simulink model "test_pi_gazebo_2023a"  (R2023a)
settings: Solver=FixedStepAuto  StartTime=0.0  StopTime=inf  RelTol=1e-3
undefined symbols (not defined in the file): angular, DiscIntNeverNeededParam, linear
libraries: ros2lib x14, robotcorelib x3, simulink x1
settings Model: Creator=johvany  LastModifiedBy=l15
settings OptimizationCC: EnhancedBackFolding=on  PassReuseOutputArgsThreshold=0  ZeroExternalMemoryAtStartup=off  ZeroInternalMemoryAtStartup=off  MaxStackSize=64  OptimizeBlockOrder=speed  DifferentSizesBufferReuse=on  OptimizationCustomize=off
settings DebuggingCC: ParameterTunabilityLossMsg=error
settings HardwareCC: ProdBitPerLong=64  ProdHWDeviceType=Intel->x86-64 (Linux 64)  UseEmbeddedCoderFeatures=off
settings SFSimCC: MATLABDynamicMemAlloc=off
settings RTWCC: Description=Embedded Coder  SystemTargetFile=ert.tlc  HardwareBoard=Robot Operating System 2 (ROS 2)  TLCOptions="-aInlineSetEventsForThisBaseRateFcn=TLC_FALSE -aSuppressMultiTaskScheduler=TLC_FALSE  -aRateBasedStepFcn=0"  TemplateMakefile=ert_default_tmf  Toolchain=Colcon Tools  TargetLang=C++
settings CodeAppCC: ForceParamTrailComments=on  OperatorAnnotations=on
settings ERTTargetCC: ERTCustomFileBanners=off  CodeInterfacePackaging=C++ class  SupportContinuousTime=on  SupportNonInlinedSFcns=on  RemoveResetFunc=off  ModelStepFunctionPrototypeControlCompliant=off  RootIOFormat=Structure reference

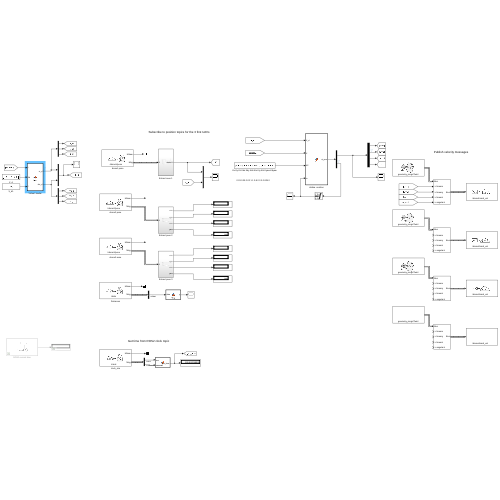
[thumbnail: Simulink's stored preview of the top-level diagram]
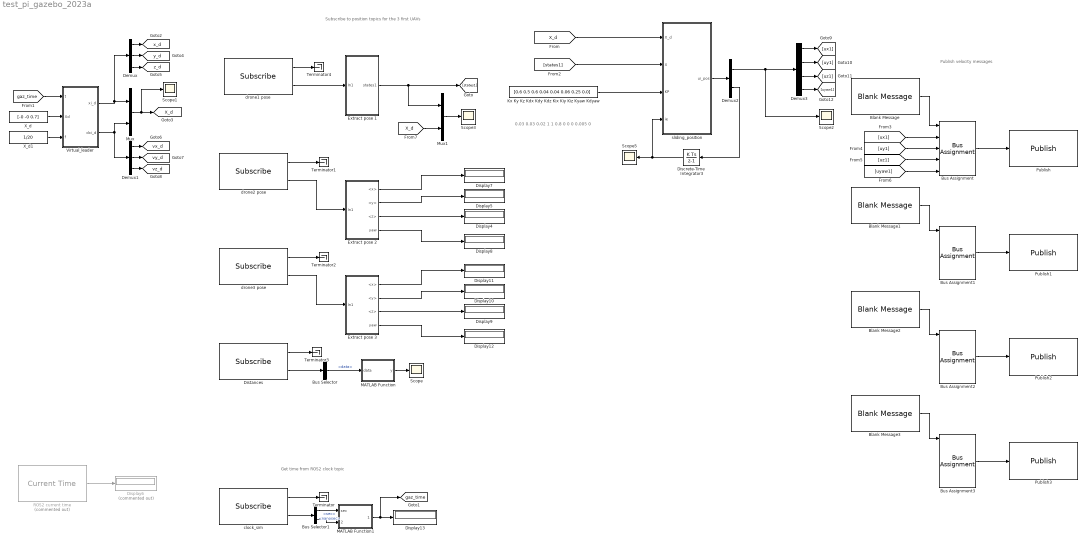
== system test_pi_gazebo_2023a ==
  note: Publish velocity messages
  note: Subscribe to position topics for the 3 first UAVs
  note: Get time from ROS2 clock topic
  note: 0.03 0.03 0.02 1 1 0.8 0 0 0 0.005 0
  Blank Message{,1..3} (4 alike) : ros2lib/Blank Message  messageClass=Message  entityType=geometry_msgs/Twist  messageType=geometry_msgs/Twist  SampleTime=inf
  Bus Assignment{,1..3} (4 alike) : BusAssignment  AssignedSignals=linear.x,linear.y,linear.z,angular.z
  Bus Selector : BusSelector  OutputSignals=data
  Bus Selector1 : BusSelector  OutputSignals=clock.sec,clock.nanosec
  Demux : Demux  Outputs=3
  Demux1 : Demux  Outputs=3
  Demux2 : Demux  Outputs=2
  Demux3 : Demux
  Discrete-Time Integrator3 : DiscreteIntegrator  SampleTime=-1  LimitOutput=on  UpperSaturationLimit=1  LowerSaturationLimit=-1  ICPrevOutput=DiscIntNeverNeededParam  ICPrevScaledInput=DiscIntNeverNeededParam
  Display{4..5,7..13} (9 alike) : Display
      Display13 settings: Decimation=4
  Display6 : Display  Commented=on
  Distances : ros2lib/Subscribe  topicSource=Select from ROS network  topic=/dists  messageType=std_msgs/Float32MultiArray  sampleTime=-1  QOSHistory=Keep last  QOSDepth=1  QOSReliability=Reliable  QOSDurability=Volatile
  Extract pose 1 : Subsystem
  Extract pose 2 : Subsystem
  Extract pose 3 : Subsystem
  Kx Ky Kz Kdx Kdy Kdz Kix Kiy Kiz Kyaw Kdyaw : Constant  Value=[0.6 0.5 0.6 0.04 0.04 0.06 0.25 0.0]
  MATLAB Function : MATLAB Function  TreatAsAtomicUnit=on
  MATLAB Function1 : MATLAB Function  TreatAsAtomicUnit=on
  Mux : Mux  Inputs=2
  Mux1 : Mux  Inputs=2
  Publish : ros2lib/Publish  topicSource=Select from ROS network  topic=/drone1/cmd_vel  messageType=geometry_msgs/Twist  QOSHistory=Keep last  QOSDepth=1  QOSReliability=Reliable  QOSDurability=Volatile
  Publish1 : ros2lib/Publish  topicSource=Select from ROS network  topic=/drone2/cmd_vel  messageType=geometry_msgs/Twist  QOSHistory=Keep last  QOSDepth=1  QOSReliability=Reliable  QOSDurability=Volatile
  Publish2 : ros2lib/Publish  topicSource=Select from ROS network  topic=/drone3/cmd_vel  messageType=geometry_msgs/Twist  QOSHistory=Keep last  QOSDepth=1  QOSReliability=Reliable  QOSDurability=Volatile
  Publish3 : ros2lib/Publish  topicSource=Select from ROS network  topic=/drone4/cmd_vel  messageType=geometry_msgs/Twist  QOSHistory=Keep last  QOSDepth=1  QOSReliability=Reliable  QOSDurability=Volatile
  ROS2 current time : ros2lib/Current Time  Commented=on  OutputFormat=double  SampleTime=-1  ModelName=test_pid_gazebo
  Scope{,1..3,5} (5 alike) : Scope
  Terminator{,1..4} (5 alike) : Terminator
  Virtual_leader : MATLAB Function  TreatAsAtomicUnit=on
  X_d : Constant  Value=[-0 -0 0.7]
  X_d1 : Constant  Value=1/20
  clock_sim : ros2lib/Subscribe  topicSource=Select from ROS network  topic=/clock  messageType=rosgraph_msgs/Clock  sampleTime=-1  QOSHistory=Keep last  QOSDepth=1  QOSReliability=Reliable  QOSDurability=Volatile
  drone1 pose : ros2lib/Subscribe  topicSource=Select from ROS network  topic=/drone1/pose  messageType=geometry_msgs/PoseStamped  sampleTime=-1  QOSHistory=Keep last  QOSDepth=1  QOSReliability=Reliable  QOSDurability=Volatile
  drone2 pose : ros2lib/Subscribe  topicSource=Select from ROS network  topic=/drone2/pose  messageType=geometry_msgs/PoseStamped  sampleTime=-1  QOSHistory=Keep last  QOSDepth=1  QOSReliability=Reliable  QOSDurability=Volatile
  drone3 pose : ros2lib/Subscribe  topicSource=Select from ROS network  topic=/drone3/pose  messageType=geometry_msgs/PoseStamped  sampleTime=-1  QOSHistory=Keep last  QOSDepth=1  QOSReliability=Reliable  QOSDurability=Volatile
  sliding_position : MATLAB Function  TreatAsAtomicUnit=on
  tag scope: X_d=global, gaz_time=global, vx_d=global, vy_d=global, vz_d=global, x_d=global, y_d=global, z_d=global
  wires:
  clock_sim/1 -> Terminator/1
  ROS2 current time/1 -> Display6/1
  Extract pose 2/3(<z>) -> Display4/1
  drone2 pose/2 -> Extract pose 2/1(In1)
  Extract pose 2/1(<x>) -> Display7/1
  Extract pose 2/4(yaw) -> Display8/1
  Extract pose 2/2(<y>) -> Display5/1
  drone2 pose/1 -> Terminator1/1
  Extract pose 3/3(<z>) -> Display9/1
  drone3 pose/2 -> Extract pose 3/1(In1)
  Extract pose 3/1(<x>) -> Display11/1
  Extract pose 3/4(yaw) -> Display12/1
  Extract pose 3/2(<y>) -> Display10/1
  drone3 pose/1 -> Terminator2/1
  Blank Message/1 -> Bus Assignment/1
  Bus Assignment/1 -> Publish/1
  Blank Message1/1 -> Bus Assignment1/1
  Bus Assignment1/1 -> Publish1/1
  Blank Message2/1 -> Bus Assignment2/1
  Bus Assignment2/1 -> Publish2/1
  Blank Message3/1 -> Bus Assignment3/1
  Bus Assignment3/1 -> Publish3/1
  Distances/1 -> Terminator3/1
  Distances/2 -> Bus Selector/1
  Bus Selector/1 -> MATLAB Function/1(data)  "<data>"
  MATLAB Function/1(y) -> Scope/1
  sliding_position/1(ui_pos) -> Demux2/1
  Discrete-Time Integrator3/1 -> Scope5/1, sliding_position/4(ie)
  [states1] -> sliding_position/2(X)
  Demux2/2 -> Discrete-Time Integrator3/1
  [X_d] -> sliding_position/1(X_d)
  clock_sim/2 -> Bus Selector1/1
  Bus Selector1/1 -> MATLAB Function1/1(sec)  "<sec>"
  Bus Selector1/2 -> MATLAB Function1/2(nanosec)  "<nanosec>"
  Demux1/1 -> [vx_d]
  Demux1/3 -> [vz_d]
  Demux/1 -> [x_d]
  Demux/2 -> [y_d]
  Virtual_leader/2(dxi_d) -> Mux/2, Demux1/1
  Mux/1 -> Scope1/1, [X_d]
  Demux1/2 -> [vy_d]
  [gaz_time] -> Virtual_leader/1(t)
  Demux/3 -> [z_d]
  Virtual_leader/1(xi_d) -> Demux/1, Mux/1
  drone1 pose/1 -> Terminator4/1
  drone1 pose/2 -> Extract pose 1/1(In1)
  MATLAB Function1/1(gaz_time) -> [gaz_time], Display13/1
  Extract pose 1/1(states1) -> Mux1/1, [states1]
  Kx Ky Kz Kdx Kdy Kdz Kix Kiy Kiz Kyaw Kdyaw/1 -> sliding_position/3(KP)
  Demux2/1 -> Scope2/1, Demux3/1
  Demux3/1 -> [ux1]
  Demux3/3 -> [uz1]
  Demux3/2 -> [uy1]
  [ux1] -> Bus Assignment/2
  [uy1] -> Bus Assignment/3
  [uz1] -> Bus Assignment/4
  [uyaw1] -> Bus Assignment/5
  X_d/1 -> Virtual_leader/2(Xd)
  Demux3/4 -> [uyaw1]
  [X_d] -> Mux1/2
  Mux1/1 -> Scope3/1
  X_d1/1 -> Virtual_leader/3(f)

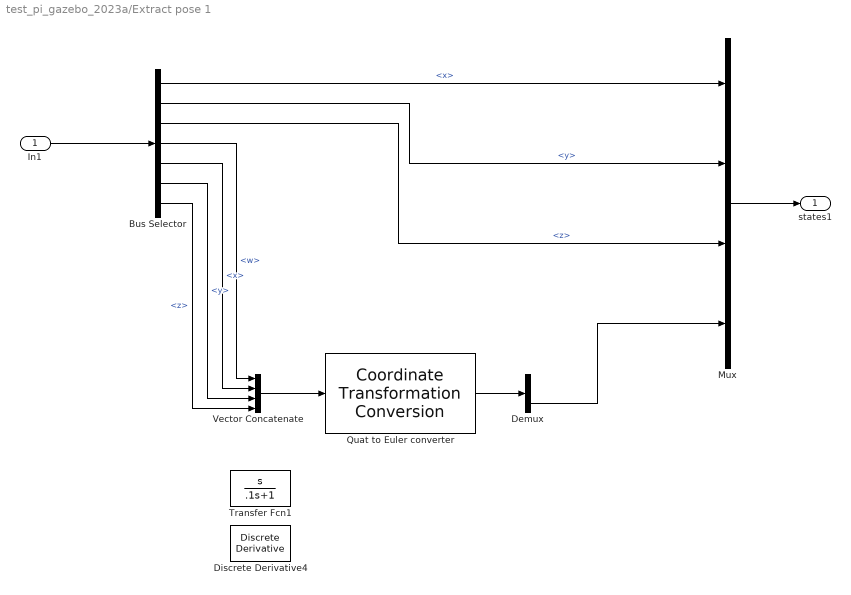
== system test_pi_gazebo_2023a/Extract pose 1 ==
  In1 : Inport
  Bus Selector : BusSelector  OutputSignals=pose.position.x,pose.position.y,pose.position.z,pose.orientation.w,pose.orientation.x,pose.orientation.y,pose.orientation.z
  Demux : Demux  Outputs=3
  Discrete Derivative4 : simulink/Discrete/Discrete Derivative  gainval=1.0  ICPrevScaledInput=0.0  OutMin=[]  OutMax=[]  OutDataType=fixdt(1, 16)  OutScaling=2^-10  DoSatur=off
  Mux : Mux
  Quat to Euler converter : robotcorelib/Coordinate Transformation Conversion  InputRepresentation=Quaternion  InputEulerSequence=ZYX  ShowTrVecInputPort=on  OutputRepresentation=Euler Angles  OutputEulerSequence=XYZ  ShowTrVecOutputPort=on  SimulateUsing=Interpreted execution
      settings: LibrarySourceBlock=roslib/Utilities/Coordinate Transformation Conversion
  Transfer Fcn1 : TransferFcn  Numerator=[1 0]  Denominator=[.1 1]
  Vector Concatenate : Concatenate  NumInputs=4
  states1 : Outport
  wires:
  Bus Selector/5 -> Vector Concatenate/2  "<x>"
  Quat to Euler converter/1 -> Demux/1
  Demux/3 -> Mux/4
  Bus Selector/6 -> Vector Concatenate/3  "<y>"
  Bus Selector/1 -> Mux/1  "<x>"
  Bus Selector/7 -> Vector Concatenate/4  "<z>"
  Vector Concatenate/1 -> Quat to Euler converter/1
  In1/1 -> Bus Selector/1
  Bus Selector/4 -> Vector Concatenate/1  "<w>"
  Bus Selector/2 -> Mux/2  "<y>"
  Bus Selector/3 -> Mux/3  "<z>"
  Mux/1 -> states1/1

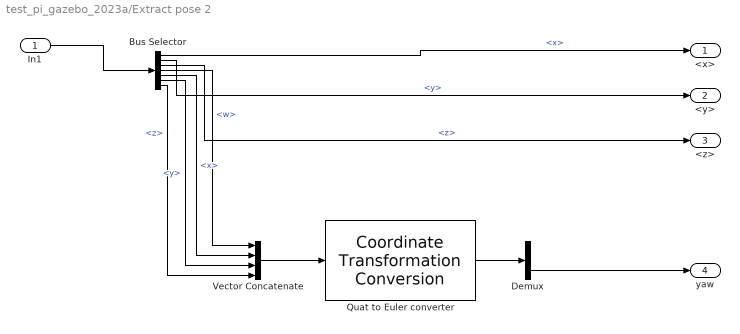
== system test_pi_gazebo_2023a/Extract pose 2 ==
  In1 : Inport
  Bus Selector : BusSelector  OutputSignals=pose.position.x,pose.position.y,pose.position.z,pose.orientation.w,pose.orientation.x,pose.orientation.y,pose.orientation.z
  Demux : Demux  Outputs=3
  Quat to Euler converter : robotcorelib/Coordinate Transformation Conversion  InputRepresentation=Quaternion  InputEulerSequence=ZYX  ShowTrVecInputPort=on  OutputRepresentation=Euler Angles  OutputEulerSequence=XYZ  ShowTrVecOutputPort=on  SimulateUsing=Interpreted execution
      settings: LibrarySourceBlock=roslib/Utilities/Coordinate Transformation Conversion
  Vector Concatenate : Concatenate  NumInputs=4
  <x> : Outport
  <y> : Outport  Port=2
  <z> : Outport  Port=3
  yaw : Outport  Port=4
  wires:
  Bus Selector/5 -> Vector Concatenate/2  "<x>"
  Quat to Euler converter/1 -> Demux/1
  Demux/3 -> yaw/1
  Bus Selector/6 -> Vector Concatenate/3  "<y>"
  Bus Selector/1 -> <x>/1  "<x>"
  Bus Selector/7 -> Vector Concatenate/4  "<z>"
  Vector Concatenate/1 -> Quat to Euler converter/1
  In1/1 -> Bus Selector/1
  Bus Selector/4 -> Vector Concatenate/1  "<w>"
  Bus Selector/2 -> <y>/1  "<y>"
  Bus Selector/3 -> <z>/1  "<z>"

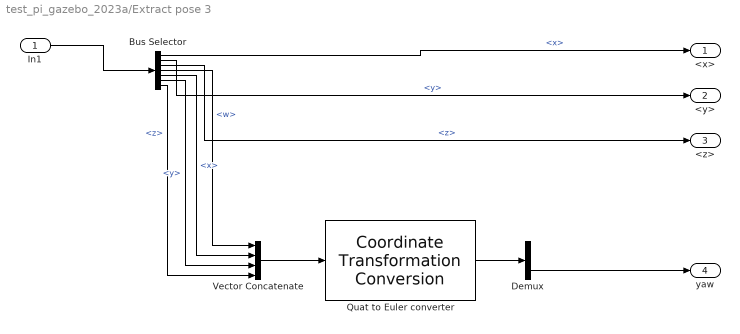
== system test_pi_gazebo_2023a/Extract pose 3 ==
  In1 : Inport
  Bus Selector : BusSelector  OutputSignals=pose.position.x,pose.position.y,pose.position.z,pose.orientation.w,pose.orientation.x,pose.orientation.y,pose.orientation.z
  Demux : Demux  Outputs=3
  Quat to Euler converter : robotcorelib/Coordinate Transformation Conversion  InputRepresentation=Quaternion  InputEulerSequence=ZYX  ShowTrVecInputPort=on  OutputRepresentation=Euler Angles  OutputEulerSequence=XYZ  ShowTrVecOutputPort=on  SimulateUsing=Interpreted execution
      settings: LibrarySourceBlock=roslib/Utilities/Coordinate Transformation Conversion
  Vector Concatenate : Concatenate  NumInputs=4
  <x> : Outport
  <y> : Outport  Port=2
  <z> : Outport  Port=3
  yaw : Outport  Port=4
  wires:
  Bus Selector/5 -> Vector Concatenate/2  "<x>"
  Quat to Euler converter/1 -> Demux/1
  Demux/3 -> yaw/1
  Bus Selector/6 -> Vector Concatenate/3  "<y>"
  Bus Selector/1 -> <x>/1  "<x>"
  Bus Selector/7 -> Vector Concatenate/4  "<z>"
  Vector Concatenate/1 -> Quat to Euler converter/1
  In1/1 -> Bus Selector/1
  Bus Selector/4 -> Vector Concatenate/1  "<w>"
  Bus Selector/2 -> <y>/1  "<y>"
  Bus Selector/3 -> <z>/1  "<z>"

== matlab function test_pi_gazebo_2023a/MATLAB Function1 ==
  data: sec input; gaz_time output; nanosec input
function gaz_time = fcn(sec, nanosec)

nanosec1 = double(nanosec)/1000000000; %*10^(-9);

sec1 = double(sec);

gaz_time = sec1 + nanosec1;

== matlab function test_pi_gazebo_2023a/MATLAB Function ==
  data: data input; y output
function y = fcn(data)

DATA = data(1:20);
d1 = DATA(1);
d2 = DATA(2);
d3 = DATA(3);
y = [d1;d2;d3];

== matlab function test_pi_gazebo_2023a/Virtual_leader ==
  data: t input; xi_d output; dxi_d output; Xd input; f input
function [xi_d, dxi_d]  = fcn(t, Xd, f)
%#codegen



%f=1/40;    %freq in Hz
radius=0.4;   %radius in meters
f2 = 1/35;
radius2 = 1;
sel=1;      %inputs or parameters dont work! only local vars ...

if sel == 1
    if t < 40
       xd     =  0;
       xdotd  =  0;
           
       yd     = 0;
       ydotd  = 0;
           
       zd     = 0.7;  
       zdotd  = 0; 
           
       xi_d =[xd; yd; zd];
       dxi_d=[xdotd; ydotd; zdotd]; 
       
    elseif t < 70
        xd     =  0.4;
        xdotd  =  0;
            
        yd     = -0.4;
        ydotd  = 0;
            
        zd     = 0.7;  
        zdotd  = 0; 
            
        xi_d =[xd; yd; zd];
        dxi_d=[xdotd; ydotd; zdotd]; 
        
    else
       xd     = radius*sin(2*pi*f*t);
       xdotd  = radius*2*pi*f*cos(2*pi*f*t);
            
       yd     = radius*cos(2*pi*f*t);
       ydotd  = -radius*2*pi*f*sin(2*pi*f*t);
            
       zd     = 0.7;  %radius*cos(2*pi*f*t) + 5;
       zdotd  = 0;  %-radius*2*pi*f*sin(2*pi*f*t);
           
       xi_d =[xd; yd; zd];
       dxi_d=[xdotd; ydotd; zdotd];
       
    end
end

 if(sel==2)
     xd     =  Xd(1);
     xdotd  =  0;
          
     yd     = Xd(2);
     ydotd  = 0;
          
     zd     = Xd(3);  
     zdotd  = 0; 
          
     xi_d =[xd; yd; zd];
     dxi_d=[xdotd; ydotd; zdotd]; 
     
 end

== matlab function test_pi_gazebo_2023a/sliding_position ==
  data: X_d input; ui_pos output; X input; KP input; ie input
function ui_pos = fcn(X_d, X, KP, ie)

%Control gains 
Kx = KP(1); Ky = KP(2); Kz = KP(3);
Kix = KP(4); Kiy = KP(5); Kiz = KP(6);
Kyaw = KP(7); Kiyaw = KP(8);

%Separation of desired and actual positions, velocities ans accelerations in their components
X_l = X_d(1:6); 
xl = X_l(1);    vxl = X_l(4);   
yl = X_l(2);    vyl = X_l(5);   
zl = X_l(3);    vzl = X_l(6);   

X_a = X(1:4);
xac = X_a(1);     
yac = X_a(2);     
zac = X_a(3);     
yaw = X_a(4);     

%Integral of the error
ieX = ie(1:4);
iex = ieX(1);
iey = ieX(2);
iez = ieX(3);
ieyaw = ieX(4);

%Errors definition (position and velocity)
ex = xl - xac;    
ey = yl - yac;    
ez = zl - zac;    
eyaw = 0 - yaw;  

%First part of the control u_o
u_ox = Kx*ex + Kix*iex;
u_oy = Ky*ey + Kiy*iey;
u_oz = Kz*ez + Kiz*iez;
ui_yaw = Kyaw*eyaw + Kiyaw*ieyaw;

ui_pos = [u_ox;u_oy;u_oz;ui_yaw;ex;ey;ez;eyaw];
